simulink library "ilcPathOpt_cl"  (R2018b)
settings: Solver=VariableStepAuto  StartTime=0.0  StopTime=10.0  RelTol=1e-3
undefined symbols (not defined in the file or in its folder): hiLvlCtrl, initializeBussesFromBlock
libraries: stopwatch_ul x2, ilcPerfIndx_cl x1, ilcPhase_cl x1, ilcUpdate_cl x1, runningAvg_ul x1
settings Model: Creator=mcobb  LastModifiedBy=mcobb

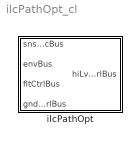
== system ilcPathOpt_cl ==
  ilcPathOpt : Subsystem  LoadFcn=initializeBussesFromBlock(gcb)  InitFcn=initializeBussesFromBlock(gcb)  StartFcn=initializeBussesFromBlock(gcb)  mask{ctrl=hiLvlCtrl}
      mask prompts: ctrl "Controller Object"
      settings: MinAlgLoopOccurrences=on

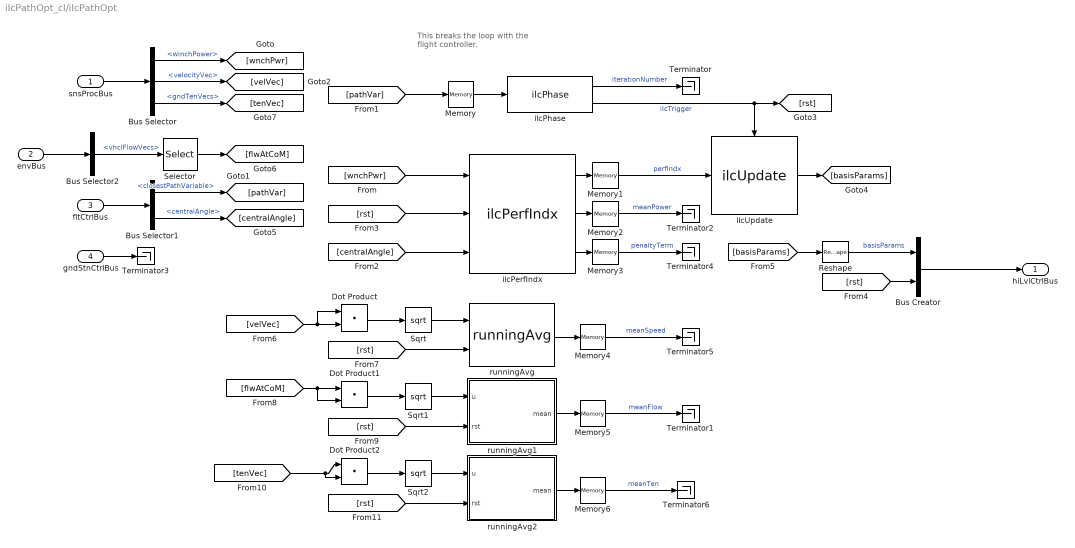
== system ilcPathOpt_cl/ilcPathOpt ==
  note: This breaks the loop
      | with the flight controller.
  snsProcBus : Inport  OutDataTypeStr=Bus: sensorsProcessingBus
  envBus : Inport  Port=2  OutDataTypeStr=Bus: envBus
  fltCtrlBus : Inport  Port=3  OutDataTypeStr=Bus: fltCtrlBus
  gndStnCtrlBus : Inport  Port=4  OutDataTypeStr=Bus: gndStnCtrlBus
  Bus Creator : BusCreator  Inputs=2  OutDataTypeStr=Bus: hiLvlCtrlBus
  Bus Selector : BusSelector  OutputSignals=winchPower,velocityVec,gndTenVecs
  Bus Selector1 : BusSelector  OutputSignals=closestPathVariable,centralAngle
  Bus Selector2 : BusSelector  OutputSignals=vhclFlowVecs
  Dot Product : DotProduct  InputSameDT=on  OutDataTypeStr=Inherit: Inherit via internal rule
  Dot Product1 : DotProduct  InputSameDT=on  OutDataTypeStr=Inherit: Inherit via internal rule
  Dot Product2 : DotProduct  InputSameDT=on  OutDataTypeStr=Inherit: Inherit via internal rule
  Memory{,1..6} (7 alike) : Memory
  Reshape : Reshape  OutputDimensionality=Row vector (2-D)
  Selector : Selector  NumberOfDimensions=2  InputPortWidth=3  IndexOptions=Select all,Index vector (dialog)  Indices=[1 3],5  OutputSizes=1,1
  Sqrt : Sqrt  SaturateOnIntegerOverflow=on
  Sqrt1 : Sqrt  SaturateOnIntegerOverflow=on
  Sqrt2 : Sqrt  SaturateOnIntegerOverflow=on
  Terminator{,1..6} (7 alike) : Terminator
  ilcPerfIndx : ilcPerfIndx_cl/ilcPerfIndx  w=ctrl.penaltyWeight.Value
  ilcPhase : ilcPhase_cl/ilcPhase  upperLim=ctrl.pathVarUpperLim.Value  lowerLim=ctrl.pathVarLowerLim.Value  numInitLaps=ctrl.numInitLaps.Value
  ilcUpdate : ilcUpdate_cl/ilcUpdate  initBasisParams=ctrl.initBasisParams.Value  lrn=ctrl.learningGain.Value  AdaptationParameter=ctrl.forgettingFactor.Value  trstRgn=ctrl.trustRegion.Value  amp=ctrl.excitationAmp.Value  enableVec=ctrl.optEnable.Value
  runningAvg : runningAvg_ul/runningAvg  SystemSampleTime=-1
  runningAvg1 : Subsystem
  runningAvg2 : Subsystem
  hiLvlCtrlBus : Outport  OutDataTypeStr=Bus: hiLvlCtrlBus
  wires:
  Memory1/1 -> ilcUpdate/1  "perfIndx"
  snsProcBus/1 -> Bus Selector/1
  envBus/1 -> Bus Selector2/1
  fltCtrlBus/1 -> Bus Selector1/1
  gndStnCtrlBus/1 -> Terminator3/1
  ilcUpdate/1 -> [basisParams]
  Bus Selector/1 -> [wnchPwr]  "<winchPower>"
  [wnchPwr] -> ilcPerfIndx/1
  Bus Selector1/1 -> [pathVar]  "<closestPathVariable>"
  [pathVar] -> Memory/1
  [rst] -> ilcPerfIndx/2
  ilcPhase/2 -> [rst], ilcUpdate/Trigger  "ilcTrigger"
  ilcPerfIndx/1 -> Memory1/1
  ilcPhase/1 -> Terminator/1  "iterationNumber"
  ilcPerfIndx/2 -> Memory2/1
  Memory2/1 -> Terminator2/1  "meanPower"
  Memory3/1 -> Terminator4/1  "penaltyTerm"
  ilcPerfIndx/3 -> Memory3/1
  [rst] -> Bus Creator/2
  [basisParams] -> Reshape/1
  Memory/1 -> ilcPhase/1
  Reshape/1 -> Bus Creator/1  "basisParams"
  Bus Selector1/2 -> [centralAngle]  "<centralAngle>"
  [centralAngle] -> ilcPerfIndx/3
  Bus Selector/2 -> [velVec]  "<velocityVec>"
  [velVec] -> Dot Product/1, Dot Product/2
  [rst] -> runningAvg/2
  runningAvg/1 -> Memory4/1
  Memory4/1 -> Terminator5/1  "meanSpeed"
  Dot Product/1 -> Sqrt/1
  Sqrt/1 -> runningAvg/1
  Bus Selector2/1 -> Selector/1  "<vhclFlowVecs>"
  Selector/1 -> [flwAtCoM]
  Sqrt1/1 -> runningAvg1/1(u)
  Dot Product1/1 -> Sqrt1/1
  Memory5/1 -> Terminator1/1  "meanFlow"
  runningAvg1/1(mean) -> Memory5/1
  [rst] -> runningAvg1/2(rst)
  [flwAtCoM] -> Dot Product1/2, Dot Product1/1
  Bus Selector/3 -> [tenVec]  "<gndTenVecs>"
  [tenVec] -> Dot Product2/2, Dot Product2/1
  [rst] -> runningAvg2/2(rst)
  runningAvg2/1(mean) -> Memory6/1
  Memory6/1 -> Terminator6/1  "meanTen"
  Dot Product2/1 -> Sqrt2/1
  Sqrt2/1 -> runningAvg2/1(u)
  Bus Creator/1 -> hiLvlCtrlBus/1

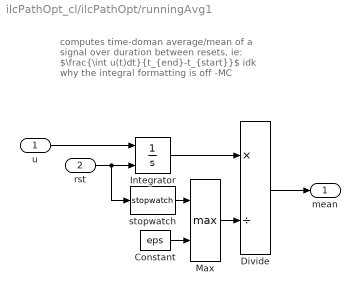
== system ilcPathOpt_cl/ilcPathOpt/runningAvg1 ==
  note: computes time-doman average/mean of a
      | signal over duration between resets, ie:
      | $\frac{\int u(t)dt}{t_{end}-t_{start}}$
      | idk why the integral formatting is off -MC
  u : Inport
  rst : Inport  Port=2
  Constant : Constant  Value=eps
  Divide : Product  Inputs=*/
  Integrator : Integrator  ExternalReset=rising
  Max : MinMax  Function=max  Inputs=2
  stopwatch : stopwatch_ul/stopwatch  SystemSampleTime=-1
  mean : Outport
  wires:
  Integrator/1 -> Divide/1
  u/1 -> Integrator/1
  stopwatch/1 -> Max/1
  Divide/1 -> mean/1
  Constant/1 -> Max/2
  Max/1 -> Divide/2
  rst/1 -> stopwatch/1, Integrator/2

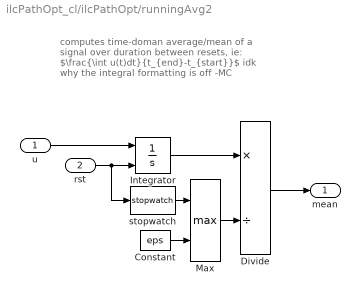
== system ilcPathOpt_cl/ilcPathOpt/runningAvg2 ==
  note: computes time-doman average/mean of a
      | signal over duration between resets, ie:
      | $\frac{\int u(t)dt}{t_{end}-t_{start}}$
      | idk why the integral formatting is off -MC
  u : Inport
  rst : Inport  Port=2
  Constant : Constant  Value=eps
  Divide : Product  Inputs=*/
  Integrator : Integrator  ExternalReset=rising
  Max : MinMax  Function=max  Inputs=2
  stopwatch : stopwatch_ul/stopwatch  SystemSampleTime=-1
  mean : Outport
  wires:
  rst/1 -> Integrator/2, stopwatch/1
  Max/1 -> Divide/2
  Constant/1 -> Max/2
  Divide/1 -> mean/1
  stopwatch/1 -> Max/1
  u/1 -> Integrator/1
  Integrator/1 -> Divide/1
